simulink library "ErrorCodeGenerator"  (R2016b)
settings: Solver=VariableStepAuto  StartTime=0.0  StopTime=10.0  RelTol=1e-3
settings Model: Creator=Nathan  LastModifiedBy=Nathan

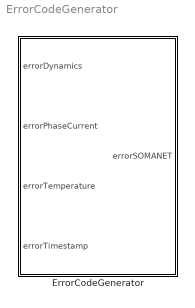
== system ErrorCodeGenerator ==
  ErrorCodeGenerator : Subsystem

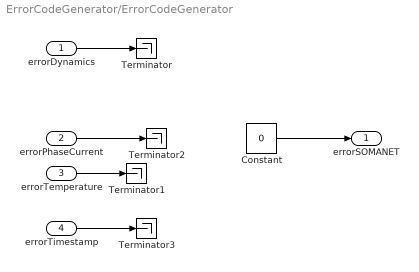
== system ErrorCodeGenerator/ErrorCodeGenerator ==
  errorDynamics : Inport
  errorPhaseCurrent : Inport  Port=2
  errorTemperature : Inport  Port=3
  errorTimestamp : Inport  Port=4
  Constant : Constant  Value=0
  Terminator{,1..3} (4 alike) : Terminator
  errorSOMANET : Outport
  wires:
  errorTimestamp/1 -> Terminator3/1
  errorDynamics/1 -> Terminator/1
  errorPhaseCurrent/1 -> Terminator2/1
  errorTemperature/1 -> Terminator1/1
  Constant/1 -> errorSOMANET/1
